simulink model "untitled"  (R2024b)
settings: Solver=VariableStepAuto  StartTime=0.0  StopTime=5000  RelTol=1e-3
values from neighbouring files (symbols this model uses):
  Cvl = Cp * rop * Vl    (= 30000)    [Lab1gpt.m]    (also in matlab.mat)
  Cvp = Cp * rop * Vp    (= 150000)    [Lab1gpt.m]    (also in matlab.mat)
  czasskok = 500    [Lab1gpt.m]    (also in matlab.mat)
  dPg = tab_Pg1(j)    [Lab1gpt.m]    (also in matlab.mat = 0.8)
  dTzew = tab_Tzew1(j)    [Lab1gpt.m]    (also in matlab.mat = 0)
  Ksl = a * Ksp    (= 173.913043478)    [Lab1gpt.m]    (also in matlab.mat)
  Ksp = Pgn / (a * (Tl_nominal - TzewN) + (Tp_nominal - TzewN))    (= 86.9565217391)    [Lab1gpt.m]    (also in matlab.mat)
  Ksw = Ksp * (Tp_nominal - TzewN) / (Tl_nominal - Tp_nominal)    (= 608.695652174)    [Lab1gpt.m]    (also in matlab.mat)
  Pg0 = tab_Pg(i)    [Lab1gpt.m]    (also in matlab.mat = 10000)
  Tl_eq = out1.Tl_eq(end)    [Lab1gpt.m]    (also in matlab.mat = 10.0117775875)
  Tp_eq = out1.Tp_eq(end)    [Lab1gpt.m]    (also in matlab.mat = 5.01437984263)
  Tzew0 = tab_Tzew(i)    [Lab1gpt.m]    (also in matlab.mat = -30)
settings Model: Creator=pawli  LastModifiedBy=Gaming PC
settings RTWCC: GPUComputeCapability=3.5

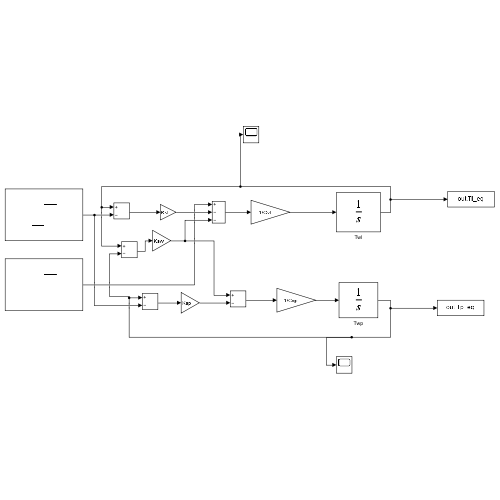
[thumbnail: Simulink's stored preview of the top-level diagram]
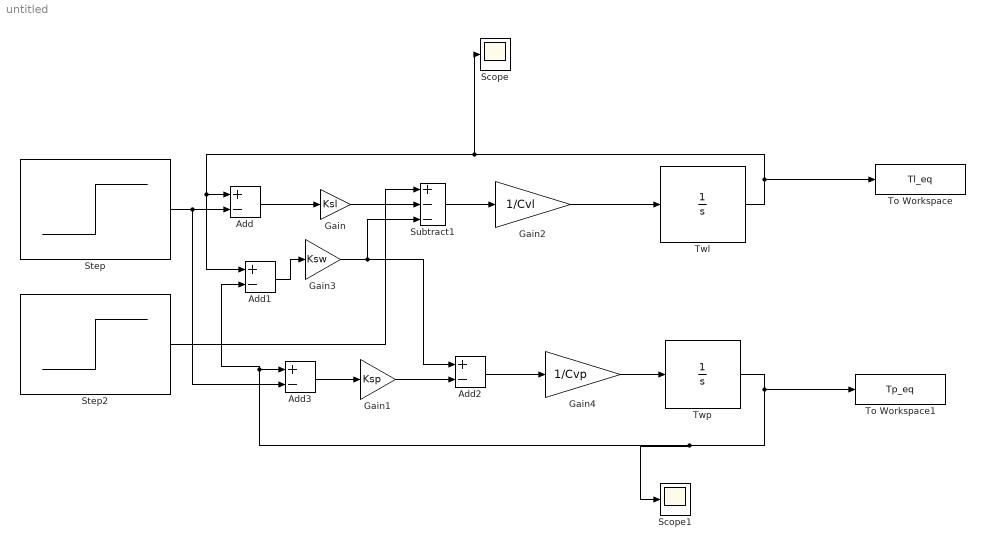
== system untitled ==
  Add{,1..3} (4 alike) : Sum  Inputs=+-
  Gain : Gain  Gain=Ksl
  Gain1 : Gain  Gain=Ksp
  Gain2 : Gain  Gain=1/Cvl
  Gain3 : Gain  Gain=Ksw
  Gain4 : Gain  Gain=1/Cvp
  Scope : Scope
  Scope1 : Scope
  Step : Step  Time=czasskok  Before=Tzew0  After=Tzew0+ dTzew  SampleTime=0
  Step2 : Step  Time=czasskok  Before=Pg0  After=Pg0 * dPg  SampleTime=0
  Subtract1 : Sum  Inputs=+--
  To Workspace : ToWorkspace  VariableName=Tl_eq  SampleTime=-1
  To Workspace1 : ToWorkspace  VariableName=Tp_eq  SampleTime=-1
  Twl : Integrator  InitialCondition=Tl_eq
  Twp : Integrator  InitialCondition=Tp_eq
  wires:
  Step/1 -> Add3/2, Add/2
  Add/1 -> Gain/1
  Gain/1 -> Subtract1/2
  Gain2/1 -> Twl/1
  Subtract1/1 -> Gain2/1
  Step2/1 -> Subtract1/1
  Gain3/1 -> Add2/1, Subtract1/3
  Add1/1 -> Gain3/1
  Gain4/1 -> Twp/1
  Add2/1 -> Gain4/1
  Add3/1 -> Gain1/1
  Gain1/1 -> Add2/2
  Twp/1 -> To Workspace1/1, Scope1/1, Add3/1, Add1/2
  Twl/1 -> To Workspace/1, Scope/1, Add1/1, Add/1
